simulink model "Hybrid2_modified"  (R2025a)
settings: Solver=FixedStepAuto  StartTime=0.0  StopTime=1.0  FixedStep=Ts  RelTol=1e-3
undefined symbols (not defined in the file or in its folder): closedLoop, controller, D1, D11, Delta, DiscIntNeverNeededParam, find_system, grid, level, protection, sensor, solarPanel, solarPlant, Ts
libraries: powerlib_extras x38, nesl_utility x29, spsSampleandHoldLib x24, spsThyristorLib x24, spsSeriesRLCBranchLib x23, simulink x22, fl_lib x18, ee_lib x12, spsEdgeDetectorLib x12, spsParallelRLCBranchLib x10, spsThreePhaseVIMeasurementLib x9, simulink_extras x8
(part 2 of 8)

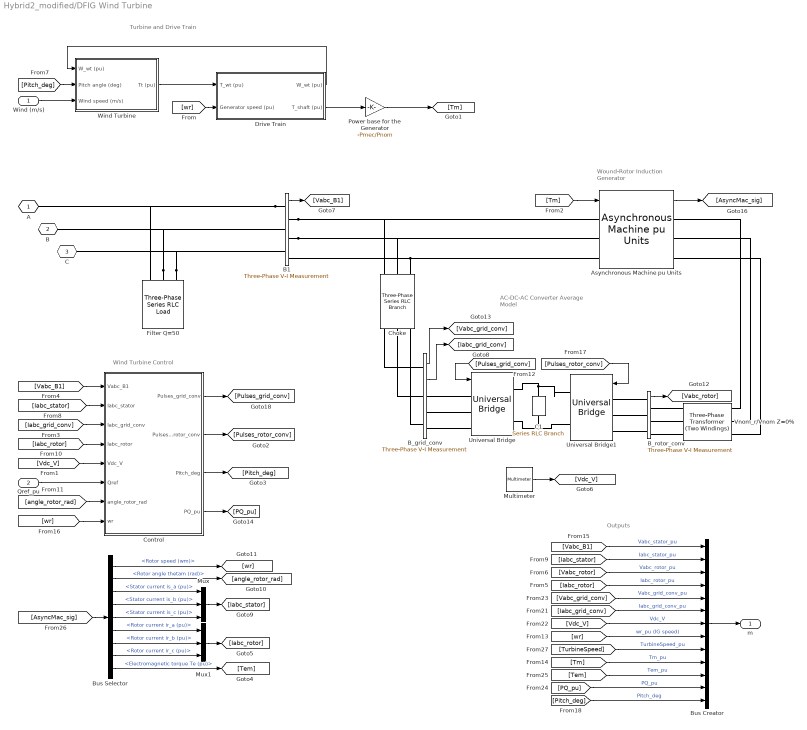
== system Hybrid2_modified/DFIG Wind Turbine ==
  note: Turbine and Drive Train
  note: Wind Turbine Control
  note: Wound-Rotor
      | Induction Generator
  note: AC-DC-AC Converter
      | Average Model
  note: Outputs
  "Wind (m/s) " : Inport
  Qref_pu : Inport  Port=2
  Asynchronous Machine pu Units : spsAsynchronousMachinepuUnitsLib/Asynchronous Machine pu Units  RotorType=Wound  PresetModel=No  MechanicalLoad=Torque Tm  ShowDetailedParameters=on  ReferenceFrame=Rotor  Units=pu  MeasurementBus=off  NominalParameters=[ Pnom Vnom Fnom ]  VoltageRatio=1  Stator=[ Rs Lls]  Rotor=[ Rr Llr]  Cage1=[0.01909 0.0397]  Cage2=[0.01909 0.0397]  Lm=Lm  Mechanical=[H F p]  PolePairs=3  InitialConditions=init  SimulateSaturation=off  Saturation="[0.212,0.4201,0.8125,1.0979,1.4799,2.2457,3.2586,4.5763,6.4763 ;   0.5,0.7,0.9,1,1.1,1.2 ,1.3,1.4,1.5]"  LoadFlowParameters=0  TsPowergui=0  TsBlock=-1  IterativeModel=Trapezoidal non iterative  IterativeDiscreteModel=Trapezoidal non iterative  Pmec=0
  B1 : spsThreePhaseVIMeasurementLib/Three-Phase V-I Measurement  VoltageMeasurement=phase-to-ground  SetLabelV=off  LabelV=Vabc  Vpu=on  VpuLL=off  CurrentMeasurement=no  SetLabelI=on  LabelI=Iabc_B1  Ipu=on  Pbase=Pnom  Vbase=Vnom  OutputType=Complex  PhasorSimulation=off  PSBequivalent=0
  B_grid_conv : spsThreePhaseVIMeasurementLib/Three-Phase V-I Measurement  VoltageMeasurement=phase-to-ground  SetLabelV=off  LabelV=Vabc_B1  Vpu=on  VpuLL=off  CurrentMeasurement=yes  SetLabelI=off  LabelI=Iabc  Ipu=on  Pbase=Pnom  Vbase=Vnom  OutputType=Complex  PhasorSimulation=off  PSBequivalent=0
  B_rotor_conv : spsThreePhaseVIMeasurementLib/Three-Phase V-I Measurement  VoltageMeasurement=phase-to-phase  SetLabelV=off  LabelV=Vabc_B1  Vpu=on  VpuLL=off  CurrentMeasurement=no  SetLabelI=off  LabelI=Iabc  Ipu=on  Pbase=Pnom  Vbase=Vnom_r  OutputType=Complex  PhasorSimulation=off  PSBequivalent=0
  Bus Creator : BusCreator  Inputs=13
  Bus Selector : BusSelector  OutputSignals=Mechanical.Rotor speed (wm),Mechanical.Rotor angle thetam (rad),Stator measurements.Stator current is_a (pu),Stator measurements.Stator current is_b (pu),Stator measurements.Stator current is_c (pu),Rotor measurements.Rotor current ir_a (pu),Rotor measurements.Rotor current ir_b (pu),Rotor measurements.Rotor current ir_c (pu),Mechanical.Electromagnetic torque Te (pu)
  C1 : spsSeriesRLCBranchLib/Series RLC Branch  LConnTagsString=__new0  RConnTagsString=__new0  BranchType=C  Resistance=[]  Inductance=[]  SetiL0=off  InitialCurrent=0  Capacitance=C_DClink  Setx0=on  InitialVoltage=Vdc_nom  Measurements=Branch voltage
  "Choke " : spsThreePhaseSeriesRLCBranchLib/Three-Phase Series RLC Branch  LConnTagsString=A|B|C  RConnTagsString=A|B|C  BranchType=RL  Resistance=R_RL*Vnom^2/Pnom  Inductance=L_RL*Vnom^2/Pnom/(2*pi*Fnom)  Capacitance=[]  Measurements=None
  Control : Subsystem
  Drive Train : Subsystem  mask(Wind Turbine shaft){H_WT=H_WT, Ksh=Ksh, D_mutual=D_mutual, wbase=2*pi*Fnom/p, w_wt0=w_wt0, torque0=torque0, Ts=Ts}
      mask prompts: H_WT "Wind turbine inertia constant H (s):"; Ksh "Shaft spring constant (pu of nominal mechanical torque/rad):"; D_mutual "Shaft mutual damping (pu of nominal mechanical torque/pu dw):"; wbase "Shaft base speed (rad/s):"; w_wt0 "Turbine initial speed (pu of base speed):"; torque0 "Initial output torque (pu of nominal mechanical torque):"; Ts "Sample time (s):"
      mask help:
      | This block implements a wind turbine drive train model. All shaft parameters are referred to high-speed shaft (generator shaft).
      |
      | The first input is the wind turbine torque in per unit (pu) based on the nominal power of the turbine and the base speed of the generator. The second input is the generator speed in pu based on the base speed of the generator.
      |
      | The outputs are:
      | 1- the transmitted torque of the shaft in pu based on the nominal power of the turbine and the base speed of the generator.
      | 2- the wind turbine speed in pu of the base speed of the generator.
  Filter Q=50 : spsThreePhaseSeriesRLCLoadLib/Three-Phase Series RLC Load  LConnTagsString=A|B|C  Configuration=Y (grounded)  NominalVoltage=Vnom  Vabc=[1e3 1e3 1e3]  Vabcp=[1e3 1e3 1e3]  NominalFrequency=Fnom  UnbalancedPower=off  ActivePower=C_var_filter/Q_filter  InductivePower=0  CapacitivePower=C_var_filter  Pabc=[10e3 9e3 11e3]  QLabc=[100 90 110]  QCabc=[100 90 110]  Pabcp=[10e3 9e3 11e3]  QLabcp=[100 90 110]  QCabcp=[100 90 110]  Measurements=None  LoadType=constant Z
  Multimeter : spsMultimeterLib/Multimeter  L=8  sel=1  yselected={}  Gain=1  OutputType=Complex  PlotAtSimulationStop=off  PhasorSimulation=off
  Mux : Mux  Inputs=3
  Mux1 : Mux  Inputs=3
  Power base for the Generator : Gain  Gain=-Pmec/Pnom  SaturateOnIntegerOverflow=on  OutDataTypeStr=Inherit: Same as input  ParamDataTypeStr=Inherit: Same as input
  Universal Bridge : spsUniversalBridgeLib/Universal Bridge  Arms=3  SnubberResistance=1e3  SnubberCapacitance=inf  Device=IGBT / Diodes  Ron=1e-4/Nb_wt  Lon=0  ForwardVoltages="[  0  0  ]"  ForwardVoltage=0  GTOparameters=[ 10e-6 , 20e-6 ]  IGBTparameters=[ 0 , 0 ]  Measurements=None  Measurements_2=None  converterType=Rectifier
  Universal Bridge1 : spsUniversalBridgeLib/Universal Bridge  Arms=3  SnubberResistance=1e3  SnubberCapacitance=inf  Device=IGBT / Diodes  Ron=1e-4/Nb_wt  Lon=0  ForwardVoltages="[  0  0  ]"  ForwardVoltage=0  GTOparameters=[ 10e-6 , 20e-6 ]  IGBTparameters=[ 0 , 0 ]  Measurements=None  Measurements_2=None  converterType=Rectifier
  Vnom_r/Vnom Z=0% : spsThreePhaseTransformerTwoWindingsLib/Three-Phase Transformer (Two Windings)  Winding1Connection=Y  Winding2Connection=Y  CoreType=Three single-phase transformers  SetSaturation=off  Hysteresis=off  DataFile='hysteresis'  SetInitialFlux=off  Measurements=None  UNITS=pu  NominalPower=[ Pnom , Fnom ]  Winding1=[ Vnom_r , 0, 0]  Winding2=[ Vnom , 0, 0]  Rm=500  Lm=inf  L0=0.5  Saturation=[ 0,0 ; 0.0024,1.2 ; 1.0,1.52 ]  InitialFluxes=[ 0.8 , -0.8 , 0.7 ]  BreakLoop=off  DiscreteSolver=Trapezoidal iterative  DataType=off  TransfoNumber=0
  Wind Turbine : Subsystem  mask(Wind Turbine){Prated=Pmec, c1_c8=c1_c8, K1_K2=K1_K2, wind0=wind0, Ts=Ts}
      mask prompts: Prated "Nominal mechanical output power (W):"; c1_c8 "Coefficients [c1 ... c8]"; K1_K2 "Parameters [K1 K2]"; wind0 "Initial wind speed (m/s):"; Ts "Sample time (s):"
      mask help:
      | This block implements a generic wind turbine models.
      |
      | The first input is the turbine speed in per unit of the generator base speed. For a synchronous or asynchronous generator, the base speed is the synchronous speed. For a permanent-magnet generator, the base speed is defined as the speed producing nominal voltage at  no load. The second input is the blade pitch angle in degrees. The third input is the wind speed in m/s.
      |
      | The output is the torque applied to the drive train in per unit based on the nominal power of the turbine and the base speed of the generator.
      mask init:
      | c1 = c1_c8(1);
      | c2 = c1_c8(2);
      | c3 = c1_c8(3);
      | c4 = c1_c8(4);
      | c5 = c1_c8(5);
      | c6 = c1_c8(6);
      | c7 = c1_c8(7);;
      | c8 = c1_c8(8);
      | 
      | K1=K1_K2(1);
      | K2=K1_K2(2);
      settings: OpenFcn=power_openblockproxy();
      mask Display: disp('');
  A : PMIOPort  Tag=PMCPort  Side=Left
  B : PMIOPort  Tag=PMCPort  Port=2  Side=Left
  C : PMIOPort  Tag=PMCPort  Port=3  Side=Left
  m : Outport  VectorParamsAs1DForOutWhenUnconnected=off
  wires:
  [Pulses_rotor_conv] -> Universal Bridge1/1
  [Pulses_grid_conv] -> Universal Bridge/1
  Multimeter/1 -> [Vdc_V]
  [Pitch_deg] -> Bus Creator/13  "Pitch_deg"
  [PQ_pu] -> Bus Creator/12  "PQ_pu"
  Control/4(PQ_pu) -> [PQ_pu]
  [Tem] -> Bus Creator/11  "Tem_pu"
  [Tm] -> Bus Creator/10  "Tm_pu"
  [TurbineSpeed] -> Bus Creator/9  "TurbineSpeed_pu"
  [Vdc_V] -> Bus Creator/7  "Vdc_V"
  [Iabc_grid_conv] -> Bus Creator/6  "Iabc_grid_conv_pu"
  [Vabc_grid_conv] -> Bus Creator/5  "Vabc_grid_conv_pu"
  [Iabc_rotor] -> Bus Creator/4  "Iabc_rotor_pu"
  [Vabc_rotor] -> Bus Creator/3  "Vabc_rotor_pu"
  [Iabc_stator] -> Bus Creator/2  "Iabc_stator_pu"
  [Vabc_B1] -> Bus Creator/1  "Vabc_stator_pu"
  Asynchronous Machine pu Units/1 -> [AsyncMac_sig]
  Control/2(Pulses_rotor_conv) -> [Pulses_rotor_conv]
  [Pitch_deg] -> Wind Turbine/2(Pitch angle (deg))
  Drive Train/1(W_wt (pu)) -> Wind Turbine/1(W_wt (pu))
  "Wind (m/s) "/1 -> Wind Turbine/3(Wind speed (m/s))
  Power base for the Generator/1 -> [Tm]
  Drive Train/2(T_shaft (pu)) -> Power base for the Generator/1
  [wr] -> Drive Train/2(Generator speed (pu))
  Wind Turbine/1(Tt (pu)) -> Drive Train/1(T_wt (pu))
  Qref_pu/1 -> Control/6(Qref)
  Bus Selector/9 -> [Tem]  "<Electromagnetic torque Te (pu)>"
  Bus Selector/1 -> [wr]  "<Rotor speed (wm)>"
  Bus Creator/1 -> m/1
  B_rotor_conv/1 -> [Vabc_rotor]
  B1/1 -> [Vabc_B1]
  [Vabc_B1] -> Control/1(Vabc_B1)
  [Iabc_grid_conv] -> Control/3(Iabc_grid_conv)
  [Iabc_rotor] -> Control/4(Iabc_rotor)
  [angle_rotor_rad] -> Control/7(angle_rotor_rad)
  Mux1/1 -> [Iabc_rotor]
  Mux/1 -> [Iabc_stator]
  [Vdc_V] -> Control/5(Vdc_V)
  Control/3(Pitch_deg) -> [Pitch_deg]
  [Iabc_stator] -> Control/2(Iabc_stator)
  [wr] -> Control/8(wr)
  Bus Selector/8 -> Mux1/3  "<Rotor current ir_c (pu)>"
  Bus Selector/7 -> Mux1/2  "<Rotor current ir_b (pu)>"
  Bus Selector/6 -> Mux1/1  "<Rotor current ir_a (pu)>"
  Bus Selector/5 -> Mux/3  "<Stator current is_c (pu)>"
  Bus Selector/4 -> Mux/2  "<Stator current is_b (pu)>"
  Bus Selector/3 -> Mux/1  "<Stator current is_a (pu)>"
  Bus Selector/2 -> [angle_rotor_rad]  "<Rotor angle thetam (rad)>"
  B_grid_conv/2 -> [Iabc_grid_conv]
  B_grid_conv/1 -> [Vabc_grid_conv]
  Control/1(Pulses_grid_conv) -> [Pulses_grid_conv]
  [AsyncMac_sig] -> Bus Selector/1
  [wr] -> Bus Creator/8  "wr_pu (IG speed)"
  [Tm] -> Asynchronous Machine pu Units/1
  connections:
  Universal Bridge1/LConn3 -- B_rotor_conv/LConn3
  Universal Bridge1/LConn2 -- B_rotor_conv/LConn2
  Universal Bridge1/LConn1 -- B_rotor_conv/LConn1
  C1/LConn1 -- Universal Bridge/RConn1 -- Universal Bridge1/RConn1
  B_grid_conv/RConn2 -- Universal Bridge/LConn2
  B_grid_conv/RConn1 -- Universal Bridge/LConn1
  B_grid_conv/RConn3 -- Universal Bridge/LConn3
  C1/RConn1 -- Universal Bridge/RConn2 -- Universal Bridge1/RConn2
  Filter Q=50/LConn3 -- B1/LConn3 -- C/RConn1
  Filter Q=50/LConn2 -- B1/LConn2 -- B/RConn1
  B1/LConn1 -- Filter Q=50/LConn1 -- A/RConn1
  B_rotor_conv/RConn3 -- Vnom_r/Vnom Z=0%/LConn3
  B_rotor_conv/RConn2 -- Vnom_r/Vnom Z=0%/LConn2
  B_rotor_conv/RConn1 -- Vnom_r/Vnom Z=0%/LConn1
  B1/RConn3 -- "Choke "/LConn3 -- Asynchronous Machine pu Units/LConn3
  B1/RConn1 -- "Choke "/LConn1 -- Asynchronous Machine pu Units/LConn1
  Asynchronous Machine pu Units/RConn3 -- Vnom_r/Vnom Z=0%/RConn3
  Asynchronous Machine pu Units/RConn1 -- Vnom_r/Vnom Z=0%/RConn1
  Asynchronous Machine pu Units/RConn2 -- Vnom_r/Vnom Z=0%/RConn2
  "Choke "/RConn3 -- B_grid_conv/LConn3
  "Choke "/RConn2 -- B_grid_conv/LConn2
  "Choke "/RConn1 -- B_grid_conv/LConn1
  B1/RConn2 -- "Choke "/LConn2 -- Asynchronous Machine pu Units/LConn2

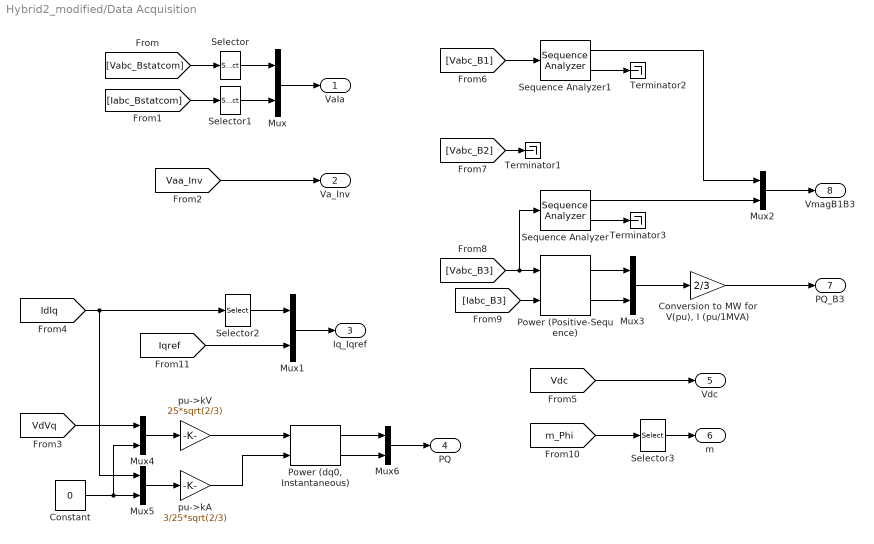
== system Hybrid2_modified/Data Acquisition ==
  Constant : Constant  Value=0
  "Conversion to MW for V(pu), I (pu/1MVA)" : Gain  Gain=2/3  SaturateOnIntegerOverflow=on  OutDataTypeStr=Inherit: Same as input  ParamDataTypeStr=Inherit: Same as input
  Mux{,1..3,6} (5 alike) : Mux  Inputs=2
  Mux4 : Mux  Inputs=[2,1]
  Mux5 : Mux  Inputs=[2,1]
  Power (Positive-Sequence) : spsPowerPositiveSequenceLib/Power (Positive-Sequence)  Freq=60  Vinit=[1, 0]  Iinit=[0, 0]  Ts=Ts
  "Power (dq0, Instantaneous)" : spsPowerdq0InstantaneousLib/Power (dq0, Instantaneous)
  Selector : Selector  InputPortWidth=3  IndexOptions=Index vector (dialog)  Indices=1  OutputSizes=1
  Selector1 : Selector  InputPortWidth=3  IndexOptions=Index vector (dialog)  Indices=1  OutputSizes=1
  Selector2 : Selector  InputPortWidth=2  IndexOptions=Index vector (dialog)  Indices=2  OutputSizes=1
  Selector3 : Selector  InputPortWidth=2  IndexOptions=Index vector (dialog)  Indices=1  OutputSizes=1
  Sequence Analyzer : spsSequenceAnalyzerLib/Sequence Analyzer  Freq=60  n=1  seq=Positive  InInit=[1, 0]  Ts=Ts
  Sequence Analyzer1 : spsSequenceAnalyzerLib/Sequence Analyzer  Freq=60  n=1  seq=Positive  InInit=[1, 0]  Ts=Ts
  Terminator1 : Terminator
  Terminator2 : Terminator
  Terminator3 : Terminator
  pu->kA : Gain  Gain=3/25*sqrt(2/3)  SaturateOnIntegerOverflow=on  OutDataTypeStr=Inherit: Same as input  ParamDataTypeStr=Inherit: Same as input
  pu->kV : Gain  Gain=25*sqrt(2/3)  SaturateOnIntegerOverflow=on  OutDataTypeStr=Inherit: Same as input  ParamDataTypeStr=Inherit: Same as input
  VaIa : Outport  VectorParamsAs1DForOutWhenUnconnected=off
  Va_Inv : Outport  Port=2  VectorParamsAs1DForOutWhenUnconnected=off
  Iq_Iqref : Outport  Port=3  VectorParamsAs1DForOutWhenUnconnected=off
  PQ : Outport  Port=4  VectorParamsAs1DForOutWhenUnconnected=off
  Vdc : Outport  Port=5  VectorParamsAs1DForOutWhenUnconnected=off
  m : Outport  Port=6  VectorParamsAs1DForOutWhenUnconnected=off
  PQ_B3 : Outport  Port=7  VectorParamsAs1DForOutWhenUnconnected=off
  VmagB1B3 : Outport  Port=8  VectorParamsAs1DForOutWhenUnconnected=off
  wires:
  [Vdc] -> Vdc/1
  Selector/1 -> Mux/1
  Selector1/1 -> Mux/2
  Mux/1 -> VaIa/1
  [m_Phi] -> Selector3/1
  [Vabc_Bstatcom] -> Selector/1
  [Iabc_Bstatcom] -> Selector1/1
  Mux1/1 -> Iq_Iqref/1
  Selector2/1 -> Mux1/1
  [Iqref] -> Mux1/2
  Selector3/1 -> m/1
  [Vaa_Inv] -> Va_Inv/1
  [Vabc_B2] -> Terminator1/1
  [Vabc_B1] -> Sequence Analyzer1/1
  Mux2/1 -> VmagB1B3/1
  Mux3/1 -> "Conversion to MW for V(pu), I (pu/1MVA)"/1
  Sequence Analyzer1/2 -> Terminator2/1
  Sequence Analyzer1/1 -> Mux2/1
  [Iabc_B3] -> Power (Positive-Sequence)/2
  [Vabc_B3] -> Sequence Analyzer/1, Power (Positive-Sequence)/1
  Sequence Analyzer/1 -> Mux2/2
  Power (Positive-Sequence)/1 -> Mux3/1
  Power (Positive-Sequence)/2 -> Mux3/2
  Sequence Analyzer/2 -> Terminator3/1
  "Conversion to MW for V(pu), I (pu/1MVA)"/1 -> PQ_B3/1
  pu->kV/1 -> "Power (dq0, Instantaneous)"/1
  pu->kA/1 -> "Power (dq0, Instantaneous)"/2
  [IdIq] -> Mux5/1, Selector2/1
  [VdVq] -> Mux4/1
  Mux4/1 -> pu->kV/1
  Mux5/1 -> pu->kA/1
  "Power (dq0, Instantaneous)"/1 -> Mux6/1
  "Power (dq0, Instantaneous)"/2 -> Mux6/2
  Mux6/1 -> PQ/1
  Constant/1 -> Mux5/2, Mux4/2

== system Hybrid2_modified/Distribution Statcom1 ==
  note: D-STATCOM
      | 25kV, +/- 3Mvar
      | Average Model
  note: +
  note: -
  note: -
  Bridge1 Average Model : spsUniversalBridgeLib/Universal Bridge  Arms=3  SnubberResistance=1e5  SnubberCapacitance=inf  Device=Average-model based VSC  Ron=1e-3  Lon=0  ForwardVoltages="[  0  0  ]"  ForwardVoltage=0  GTOparameters=[ 10e-6 , 20e-6 ]  IGBTparameters=[ 1e-6 , 2e-6 ]  Measurements=None  Measurements_2=None  converterType=Rectifier
  Bridge2 Average Model : spsUniversalBridgeLib/Universal Bridge  Arms=3  SnubberResistance=1e5  SnubberCapacitance=inf  Device=Average-model based VSC  Ron=1e-3  Lon=0  ForwardVoltages="[  0  0  ]"  ForwardVoltage=0  GTOparameters=[ 10e-6 , 20e-6 ]  IGBTparameters=[ 1e-6 , 2e-6 ]  Measurements=None  Measurements_2=None  converterType=Rectifier
  Ca_DVR : spsSeriesRLCBranchLib/Series RLC Branch  LConnTagsString=__new0  RConnTagsString=__new0  BranchType=RC  Resistance=100e-6*(2*pi*60)/40  Inductance=1.0  SetiL0=off  InitialCurrent=0  Capacitance=100e-6  Setx0=off  InitialVoltage=0  Measurements=None
  Ca_DVR1 : spsSeriesRLCBranchLib/Series RLC Branch  LConnTagsString=__new0  RConnTagsString=__new0  BranchType=RC  Resistance=100e-6*(2*pi*60)/40  Inductance=1.0  SetiL0=off  InitialCurrent=0  Capacitance=100e-6  Setx0=off  InitialVoltage=0  Measurements=None
  Ca_DVR2 : spsSeriesRLCBranchLib/Series RLC Branch  LConnTagsString=__new0  RConnTagsString=__new0  BranchType=RC  Resistance=100e-6*(2*pi*60)/40  Inductance=1.0  SetiL0=off  InitialCurrent=0  Capacitance=100e-6  Setx0=off  InitialVoltage=0  Measurements=None
  DC Link : spsParallelRLCBranchLib/Parallel RLC Branch  LConnTagsString=a  RConnTagsString=__new0  BranchType=C  Resistance=1.0  Inductance=1.0  SetiL0=off  InitialCurrent=0  Capacitance=10000e-6  Setx0=off  InitialVoltage=0  Measurements=None
  D_statcom_avg Controller : Subsystem  mask(D-STATCOM Controller){ModeOper=Voltage regulation, Vac_Ref=1.0, Qref=0, Vdc_Ref=2400, Par_VacReg=[0.55 2500], Par_VdcReg=[0.001 0.15], Par_IReg=[0.8 200 0], Ts=2e-4}
      mask prompts: ModeOper "Mode of operation:"; Vac_Ref "AC voltage setpoint Vref (pu):"; Qref "Manual mode: Qref (Reactive power in pu):"; Vdc_Ref "DC Voltage setpoint (Volts)"; Par_VacReg "Vac Regulator Gains: [ Kp  Ki ]"; Par_VdcReg "Vdc Regulator Gains: [ Kp  Ki ]"; Par_IReg "Current Regulators Gain: [ Kp Ki Kd ]"; Ts "Sample time (s)"
      mask init:
      | Kp_I=Par_IReg(1);
      | Ki_I=Par_IReg(2);
      | Kd_I=Par_IReg(3);
      | Kp_Vdc=Par_VdcReg(1);
      | Ki_Vdc=Par_VdcReg(2);
      | Kp_Vac=Par_VacReg(1);
      | Ki_Vac=Par_VacReg(2);
      mask TypeOptions ModeOper: Voltage regulation | Q regulation
  Gain : Gain  Gain=-1
  Ground : spsGroundLib/Ground  LConnTagsString=a
  Ground1 : spsGroundLib/Ground  LConnTagsString=a
  Ground2 : spsGroundLib/Ground  LConnTagsString=a
  La_DVR : spsSeriesRLCBranchLib/Series RLC Branch  LConnTagsString=__new0  RConnTagsString=__new0  BranchType=L  Resistance=1.0  Inductance=800e-6  SetiL0=off  InitialCurrent=0  Capacitance=1.0  Setx0=off  InitialVoltage=0  Measurements=None
  La_DVR1 : spsSeriesRLCBranchLib/Series RLC Branch  LConnTagsString=__new0  RConnTagsString=__new0  BranchType=L  Resistance=1.0  Inductance=800e-6  SetiL0=off  InitialCurrent=0  Capacitance=1.0  Setx0=off  InitialVoltage=0  Measurements=None
  La_DVR2 : spsSeriesRLCBranchLib/Series RLC Branch  LConnTagsString=__new0  RConnTagsString=__new0  BranchType=L  Resistance=1.0  Inductance=800e-6  SetiL0=off  InitialCurrent=0  Capacitance=1.0  Setx0=off  InitialVoltage=0  Measurements=None
  Tr A : spsLinearTransformerLib/Linear Transformer  UNITS=pu  NominalPower=[3e6/3 60]  winding1=[1250 0.03/30 0.03]  winding2=[25e3/sqrt(3) 0.03/30 0.03]  ThreeWindings=off  winding3=[60e3 0.005 0.02]  RmLm=[200 200]  Measurements=None  DataType=off
  Tr B : spsLinearTransformerLib/Linear Transformer  UNITS=pu  NominalPower=[3e6/3 60]  winding1=[1250 0.03/30 0.03]  winding2=[25e3/sqrt(3) 0.03/30 0.03]  ThreeWindings=off  winding3=[60e3 0.005 0.02]  RmLm=[200 200]  Measurements=None  DataType=off
  Tr C : spsLinearTransformerLib/Linear Transformer  UNITS=pu  NominalPower=[3e6/3 60]  winding1=[1250 0.03/30 0.03]  winding2=[25e3/sqrt(3) 0.03/30 0.03]  ThreeWindings=off  winding3=[60e3 0.005 0.02]  RmLm=[200 200]  Measurements=None  DataType=off
  Voltage Measurement : spsVoltageMeasurementLib/Voltage Measurement  Tag=PoWeRsYsTeMmEaSuReMeNt  PhasorSimulation=off  OutputType=Magnitude  PSBequivalent=0
  Voltage Measurement1 : spsVoltageMeasurementLib/Voltage Measurement  Tag=PoWeRsYsTeMmEaSuReMeNt  PhasorSimulation=off  OutputType=Magnitude  PSBequivalent=0
  A : PMIOPort  Side=Right
  B : PMIOPort  Port=2  Side=Right
  C : PMIOPort  Port=3  Side=Right
  tag scope: Vaa_Inv=global, Vdc_Statcom=global
  wires:
  [Vabc_Bstatcom] -> D_statcom_avg Controller/2(Vabc)
  [Iabc_Bstatcom] -> D_statcom_avg Controller/3(Iabc)
  Voltage Measurement/1 -> [Vdc_Statcom]
  [Vdc] -> D_statcom_avg Controller/1(Vdc)
  D_statcom_avg Controller/1(Vref_abc) -> Bridge1 Average Model/1, Gain/1
  Gain/1 -> Bridge2 Average Model/1
  Voltage Measurement1/1 -> [Vaa_Inv]
  connections:
  Bridge2 Average Model/LConn2 -- Ca_DVR1/LConn1 -- Tr B/LConn2
  Tr C/LConn2 -- Ca_DVR2/LConn1 -- Bridge2 Average Model/LConn3
  Ca_DVR1/RConn1 -- La_DVR1/RConn1 -- Tr B/LConn1
  Ca_DVR2/RConn1 -- La_DVR2/RConn1 -- Tr C/LConn1
  Tr A/LConn1 -- La_DVR/RConn1 -- Ca_DVR/RConn1
  Tr C/RConn2 -- Ground2/LConn1
  Tr B/RConn2 -- Ground1/LConn1
  Tr A/RConn2 -- Ground/LConn1
  A/RConn1 -- Tr A/RConn1
  Tr B/RConn1 -- B/RConn1
  C/RConn1 -- Tr C/RConn1
  Tr A/LConn2 -- Ca_DVR/LConn1 -- Bridge2 Average Model/LConn1 -- Voltage Measurement1/LConn2
  Bridge1 Average Model/RConn1 -- Bridge2 Average Model/RConn1 -- DC Link/LConn1 -- Voltage Measurement/LConn1
  Bridge1 Average Model/LConn1 -- La_DVR/LConn1 -- Voltage Measurement1/LConn1
  Bridge1 Average Model/LConn2 -- La_DVR1/LConn1
  Bridge1 Average Model/LConn3 -- La_DVR2/LConn1
  DC Link/RConn1 -- Bridge1 Average Model/RConn2 -- Bridge2 Average Model/RConn2 -- Voltage Measurement/LConn2

== system Hybrid2_modified/Filter & AC Measurements ==
  Current Sensor Dynamics : Subsystem
  Current Sensor1 : ee_lib/Sensors & Transducers/Current Sensor (Three-Phase)
  Neutral Port (Three-Phase) : ee_lib/Connectors & References/Neutral Port (Three-Phase)  G_parasitic=1e-12 1/Ohm
      settings: InternalSimscapePortConfiguration="{\"Bottom\":[],\"Left\":[{\"id\":\"N\",\"label\":\"~\",\"type\":\"foundation.electrical.three_phase\"}],\"Right\":[{\"id\":\"n\",\"label\":\"n\",\"type\":\"foundation.electrical.electrical\"}],\"Top\":[]}"
  PS-Simulink Converter : nesl_utility/PS-Simulink Converter  PhysicalDomain=network_engine_domain  SubClassName=ps_output  LeftPortType=input  RightPortType=output  PseudoPeriodic=off  Frequencies=[]  VectorFormat=1-D array  Unit=inherit  AffineConversion=off
  PS-Simulink Converter1 : nesl_utility/PS-Simulink Converter  PhysicalDomain=network_engine_domain  SubClassName=ps_output  LeftPortType=input  RightPortType=output  PseudoPeriodic=off  Frequencies=[]  VectorFormat=1-D array  Unit=inherit  AffineConversion=off
  Phase Voltage Sensor (Three-Phase) : ee_lib/Sensors & Transducers/Phase Voltage Sensor (Three-Phase)
  RLC (Three-Phase) : ee_lib/Passive/RLC Assemblies/RLC (Three-Phase)  port_option=ee.enum.threePhasePort.composite  component_structure=4  R=solarPlant.inductorResistance Ohm  L=solarPlant.lineInductance H  C=1e-6 F  R_parasitic=1e-6 Ohm  G_parasitic=1e-6 1/Ohm  IL_specify=on  IL_priority=High  IL=[0, 0, 0] A  IL_nominal_specify=off  IL_nominal_value=1  IL_nominal_unit=A  VC_specify=on  VC_priority=High  VC=[0, 0, 0] V  VC_nominal_specify=off  VC_nominal_value=1  VC_nominal_unit=V
      settings: InternalSimscapePortConfiguration="{\"Bottom\":[],\"Left\":[{\"id\":\"N1\",\"label\":\"~1\",\"type\":\"foundation.electrical.three_phase\"}],\"Right\":[{\"id\":\"N2\",\"label\":\"~2\",\"type\":\"foundation.electrical.three_phase\"}],\"Top\":[]}"
  Scope : Scope  NumInputPorts=2
      settings: ActiveDisplayYMinimum=-169.31893  ActiveDisplayYMaximum=165.34576
  Voltage Sensor Dynamics : Subsystem
  ABC1 : PMIOPort  Side=Left
  ABC2 : PMIOPort  Port=2  Side=Right
  N : PMIOPort  Port=3  Side=Right
  Iabc : Outport
  Vabc : Outport  Port=2
  wires:
  PS-Simulink Converter/1 -> Scope/1, Current Sensor Dynamics/1(Iabc1)
  Current Sensor Dynamics/1(Iabc2) -> Iabc/1
  Voltage Sensor Dynamics/1(Vabc2) -> Vabc/1
  PS-Simulink Converter1/1 -> Scope/2, Voltage Sensor Dynamics/1(Vabc1)
  connections:
  Current Sensor1/LConn1 -- RLC (Three-Phase)/RConn1
  Phase Voltage Sensor (Three-Phase)/LConn1 -- ABC2/RConn1 -- Current Sensor1/RConn2
  PS-Simulink Converter/LConn1 -- Current Sensor1/RConn1
  PS-Simulink Converter1/LConn1 -- Phase Voltage Sensor (Three-Phase)/RConn1
  Neutral Port (Three-Phase)/LConn1 -- Phase Voltage Sensor (Three-Phase)/RConn2
  Neutral Port (Three-Phase)/RConn1 -- N/RConn1
  RLC (Three-Phase)/LConn1 -- ABC1/RConn1

== system Hybrid2_modified/Grid ==
  Resistor : fl_lib/Electrical/Electrical Elements/Resistor  R=50 Ohm  i_specify=off  i_priority=None  i=0 A  i_nominal_specify=off  i_nominal_value=1  i_nominal_unit=A  v_specify=off  v_priority=None  v=0 V  v_nominal_specify=off  v_nominal_value=1  v_nominal_unit=V
  Voltage Source (Three-Phase) : ee_lib/Sources/Voltage Source (Three-Phase)  vline_rms=grid.actualLineVoltage V  shift=0 deg  freq=grid.frequency Hz  impedance_option=0  SShortCircuit=1e6 V*A  XR=15  R=0.01 Ohm  L=3.97e-4 H  harmonic_option=0  harmonic_orders=[5, 7, 11, 13]  harmonic_ratios=[.1, .1, .1, .1]  G_parasitic=0 1/Ohm  I_specify=off  I_priority=None  I=[ 0 0 0 ] A  I_nominal_specify=off  I_nominal_value=1  I_nominal_unit=A
  ABC : PMIOPort  Side=Left
  N : PMIOPort  Port=2  Side=Left
  E : PMIOPort  Port=3  Side=Left
  connections:
  E/RConn1 -- Resistor/RConn1
  ABC/RConn1 -- Voltage Source (Three-Phase)/RConn1
  Voltage Source (Three-Phase)/LConn1 -- N/RConn1 -- Resistor/LConn1

== system Hybrid2_modified/Linearization I//O points ==
  u2 : Inport
  u1 : Inport  Port=2
  "Set to 1 for closed-loop operation, and set to 0 when linearizing" : Gain  Gain=closedLoop  SaturateOnIntegerOverflow=on  OutDataTypeStr=Inherit: Same as input  ParamDataTypeStr=Inherit: Same as input
  Sum1 : Sum  Inputs=++|  InputSameDT=on  SaturateOnIntegerOverflow=on  OutDataTypeStr=Inherit: Same as first input
  y2 : Outport  VectorParamsAs1DForOutWhenUnconnected=off
  y1 : Outport  Port=2  VectorParamsAs1DForOutWhenUnconnected=off
  wires:
  Sum1/1 -> y1/1
  u2/1 -> Sum1/1
  "Set to 1 for closed-loop operation, and set to 0 when linearizing"/1 -> Sum1/2
  u1/1 -> y2/1, "Set to 1 for closed-loop operation, and set to 0 when linearizing"/1

== system Hybrid2_modified/MPPT ==
  Ipv : Inport
  Vpv : Inport  Port=2
  Constant : Constant  Value=solarPlant.endMPPTValue
  MPPT Algorithm : Subsystem  Variant=on
  Switch : Switch  Threshold=solarPlant.endMPPTValue  SaturateOnIntegerOverflow=off  InputSameDT=off
  Vmpp : Outport  VectorParamsAs1DForOutWhenUnconnected=off
  tag scope: Ipvnow=global, Vpvnow=global
  wires:
  Vpv/1 -> [Vpvnow], MPPT Algorithm/2(Vpv)
  Ipv/1 -> [Ipvnow], MPPT Algorithm/1(Ipv)
  Constant/1 -> Switch/1
  MPPT Algorithm/1(Vmpp) -> Switch/3, Switch/2
  Switch/1 -> Vmpp/1

== system Hybrid2_modified/Modulation Signal ==
  Vd : Inport
  Vq : Inport  Port=2
  Angle : Inport  Port=3
  Vdc : Inport  Port=4
  Gating Signal : Subsystem
  "dq to alpha beta " : Subsystem
  mabc : Outport  VectorParamsAs1DForOutWhenUnconnected=off
  wires:
  Gating Signal/1(mabc) -> mabc/1
  Vdc/1 -> Gating Signal/2(Vdc)
  "dq to alpha beta "/1(Vabc) -> Gating Signal/1(Vmod)
  Vd/1 -> "dq to alpha beta "/1("d ")
  Angle/1 -> "dq to alpha beta "/3(angle)
  Vq/1 -> "dq to alpha beta "/2(q)

== system Hybrid2_modified/PLL and Protection ==
  Vabc : Inport
  Vpv : Inport  Port=2
  Iabc : Inport  Port=3
  Constant : Constant  Value=pi/2
  Gain2 : Gain  Gain=2*pi
  Protection : Subsystem
  "Sinusoidal Measurement (PLL, Three-Phase)" : eeSinusoidalMeasurement/Sinusoidal Measurement (PLL, Three-Phase)  Kp_LF=0.05  Ki_LF=1  F0=grid.frequency  Theta0=0  Ts=0
  Subtract : Sum  Inputs=-+
  Vphm to Vsd : Gain  Gain=3/2
  w : Outport  VectorParamsAs1DForOutWhenUnconnected=off
  angle : Outport  Port=2  VectorParamsAs1DForOutWhenUnconnected=off
  Vsd : Outport  Port=3  VectorParamsAs1DForOutWhenUnconnected=off
  TripSig : Outport  Port=4  VectorParamsAs1DForOutWhenUnconnected=off
  wires:
  "Sinusoidal Measurement (PLL, Three-Phase)"/3 -> Vphm to Vsd/1
  Gain2/1 -> Protection/1(w), w/1
  "Sinusoidal Measurement (PLL, Three-Phase)"/1 -> Gain2/1
  Vabc/1 -> "Sinusoidal Measurement (PLL, Three-Phase)"/1
  Protection/1(TS) -> TripSig/1
  Vpv/1 -> Protection/3(Vpv)
  Iabc/1 -> Protection/4(Iac)
  Subtract/1 -> angle/1
  "Sinusoidal Measurement (PLL, Three-Phase)"/2 -> Subtract/2
  Constant/1 -> Subtract/1
  Vphm to Vsd/1 -> Vsd/1, Protection/2(Vsd)

== system Hybrid2_modified/Power Circuit ==
  note: Solar panel parasitic capacitance
  note: Solar panel parasitic capacitance
  C1 : fl_lib/Electrical/Electrical Elements/Capacitor  c=solarPlant.capacitance*2 F  r=1e-6 Ohm  g=0 1/Ohm  i_specify=off  i_priority=High  i=0 A  i_nominal_specify=off  i_nominal_value=1  i_nominal_unit=A  v_specify=off  v_priority=High  v=0 V  v_nominal_specify=off  v_nominal_value=1  v_nominal_unit=V  vc_specify=on  vc_priority=High  vc=solarPlant.DCMPPTValue/2 V  vc_nominal_specify=off  vc_nominal_value=1  vc_nominal_unit=V
  C2 : fl_lib/Electrical/Electrical Elements/Capacitor  c=solarPlant.capacitance*2 F  r=1e-6 Ohm  g=0 1/Ohm  i_specify=off  i_priority=High  i=0 A  i_nominal_specify=off  i_nominal_value=1  i_nominal_unit=A  v_specify=off  v_priority=High  v=0 V  v_nominal_specify=off  v_nominal_value=1  v_nominal_unit=V  vc_specify=on  vc_priority=High  vc=solarPlant.DCMPPTValue/2 V  vc_nominal_specify=off  vc_nominal_value=1  vc_nominal_unit=V
  C3 : fl_lib/Electrical/Electrical Elements/Capacitor  c=solarPlant.parasiticCapacitance/2 F  r=1 Ohm  g=0 1/Ohm  i_specify=off  i_priority=High  i=0 A  i_nominal_specify=off  i_nominal_value=1  i_nominal_unit=A  v_specify=off  v_priority=High  v=0 V  v_nominal_specify=off  v_nominal_value=1  v_nominal_unit=V  vc_specify=on  vc_priority=High  vc=solarPlant.DCMPPTValue V  vc_nominal_specify=off  vc_nominal_value=1  vc_nominal_unit=V
  C4 : fl_lib/Electrical/Electrical Elements/Capacitor  c=solarPlant.parasiticCapacitance/2 F  r=1 Ohm  g=0 1/Ohm  i_specify=off  i_priority=High  i=0 A  i_nominal_specify=off  i_nominal_value=1  i_nominal_unit=A  v_specify=off  v_priority=High  v=0 V  v_nominal_specify=off  v_nominal_value=1  v_nominal_unit=V  vc_specify=on  vc_priority=High  vc=solarPlant.DCMPPTValue V  vc_nominal_specify=off  vc_nominal_value=1  vc_nominal_unit=V
  DC Current Sensor : Subsystem
      mask Display: disp('i')
  DC Voltage Sensor : Subsystem
      mask Display: disp('v');
  Power Circuit : Subsystem  Variant=on  VariantControl=Variant1
  + : PMIOPort  Side=Left
  - : PMIOPort  Port=2  Side=Left
  ABC : PMIOPort  Port=3  Side=Right
  E : PMIOPort  Port=4  Side=Right
  wires:
  [mABC] -> Power Circuit/1(m)
  [TripSig] -> Power Circuit/2(TripSig)
  connections:
  -/RConn1 -- DC Voltage Sensor/LConn1 -- C4/LConn1 -- Power Circuit/LConn3 -- C2/RConn1
  C2/LConn1 -- Power Circuit/LConn2 -- C1/RConn1
  DC Current Sensor/LConn1 -- C3/LConn1 -- Power Circuit/LConn1 -- C1/LConn1 -- DC Voltage Sensor/RConn1
  DC Current Sensor/RConn1 -- +/RConn1
  C3/RConn1 -- E/RConn1 -- C4/RConn1
  ABC/RConn1 -- Power Circuit/RConn1

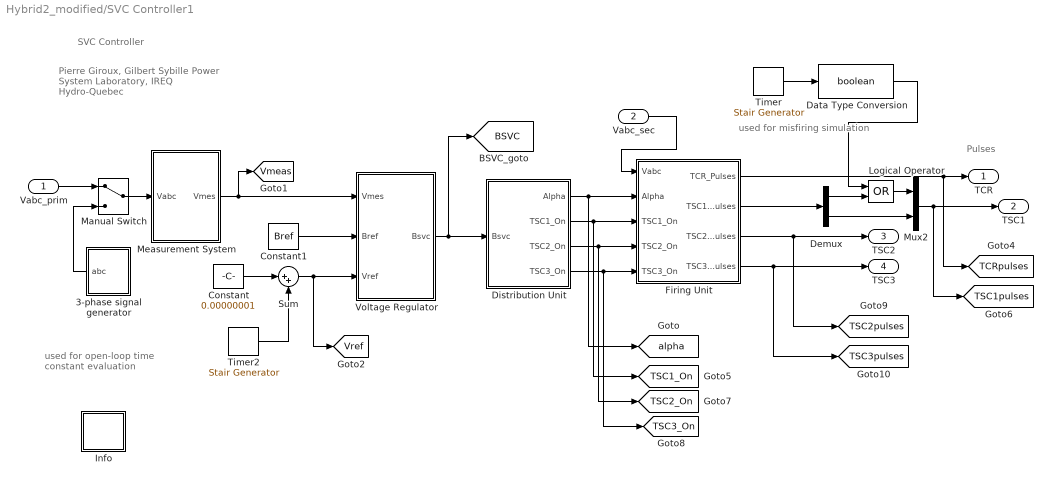
== system Hybrid2_modified/SVC Controller1 ==
  note: Pulses
  note: SVC Controller
  note: Pierre Giroux, Gilbert Sybille
      | Power System Laboratory, IREQ
      | Hydro-Quebec
  note: used for misfiring
      | simulation
  note: used for open-loop
      | time constant evaluation
  Vabc_prim : Inport  PortDimensions=3
  Vabc_sec : Inport  Port=2  PortDimensions=3
  3-phase signal generator : Subsystem
  Constant : Constant  Value=0.00000001
  Constant1 : Constant  Value=Bref
  Data Type Conversion : DataTypeConversion  OutDataTypeStr=boolean  SaturateOnIntegerOverflow=off  RndMeth=Floor
  Demux : Demux  Outputs=[1 5]
      settings: DisplayOption=none
  Distribution Unit : Subsystem  mask(Distribution Unit){ParNom=[333e6 60], Xf_xfo=0.15, Vsec_svc=16e3, L_TCR=18.7e-3, C_TSC=308.4e-6, L_TSC=1.13e-3, hyst_svc=0.1, Ts=Ts}
      mask prompts: ParNom "Transformer nominal power and frequency: [  P (VA)    Freq (Hz)  ]"; Xf_xfo "Transformer total leakage (pu/Pnom):"; Vsec_svc "Nominal secondary voltage (Volts rms ph-ph):"; L_TCR "TCR branch inductance (H):"; C_TSC "TSC branch capacitance (F):"; L_TSC "TSC branch inductance (H)"; hyst_svc "Hysteresis - Distribution unit (pu/100MVA):"; Ts "Sample time:"
      mask init:
      | Pnom_xfo=ParNom(1);
      | Freq=ParNom(2);
      | Bsec_pu100=100e6/Vsec_svc/Vsec_svc/3;
      | w=2*pi*Freq;
      | Bpu_TCR=-1/L_TCR/w/Bsec_pu100;
      | Bpu_TSC=1/(1/w/C_TSC-L_TSC*w)/Bsec_pu100;
      | B=1:-0.0025:0.0;
      | B=B';
      | for i=1:401,
      |       if B(i) <= 0,
      | 	ang = 0;
      |       elseif B(i) >= 1,
      | 	ang = pi;
      |       else,
      | 	a = pi; e = .0001;
      | 	da = a;
      | 	while abs(da)>e,
      | 		da = (pi*B(i)-a+sin(a))/(1-cos(a));
      | 		a = a + da;
      | 	end;
      | 	ang = a;
      |       end;
      |       A(i)=(180-ang*180/pi)/2+90;
      | end
      | A=A';
      | B=-B;
  Firing Unit : Subsystem  mask(Firing Unit){FiringMode=Synchronized, Nstep=0, ParInit=[0 60], Ts=Ts}
      mask prompts: FiringMode "Firing mode"; Nstep "Total delay (in number of time step)"; ParInit "Initial phase and frequency of input: [ Phase (degree)  Freq (Hz) ]"; Ts "Sample time:"
      mask init:
      | PhaseInit=ParInit(1);
      | FreqInit=ParInit(2);
      mask TypeOptions FiringMode: Synchronized | Continuous
  Info : Subsystem
      mask Display: disp('?')
  Logical Operator : Logic  Operator=OR
  Manual Switch : ManualSwitch
  Measurement System : Subsystem  mask(SVC measurement system){Vnom=735e3, ParI=[735e3*0.9998 0 60], Ts=Ts}
      mask prompts: Vnom "Nominal voltage (volts rms ph-ph)"; ParI "Initial input: [ Mag (volts rms ph-ph)  Phase (degree) Freq (Hz) ]"; Ts "Sample time:"
      mask init:
      | Mag_Init=ParI(1)/Vnom;
      | Phase_Init=ParI(2);
      | Freq_Init=ParI(3);
  Mux2 : Mux  Inputs=[1 5]
  Sum : Sum  Inputs=|++  SaturateOnIntegerOverflow=on
  Timer : spsStairGeneratorLib/Stair Generator  t="[ 0  0.121  0.121+eps ]*100"  e="[0  1  0 ]"  Ts=Ts
  Timer2 : spsStairGeneratorLib/Stair Generator  t="[ 0  0.4  0.6 ]"  e=[1 1 1 ]  Ts=Ts
  Voltage Regulator : Subsystem
  TCR : Outport  VectorParamsAs1DForOutWhenUnconnected=off
  TSC1 : Outport  Port=2  VectorParamsAs1DForOutWhenUnconnected=off
  TSC2 : Outport  Port=3  VectorParamsAs1DForOutWhenUnconnected=off
  TSC3 : Outport  Port=4  VectorParamsAs1DForOutWhenUnconnected=off
  tag scope: BSVC=global, TCRpulses=global, TSC1_On=global, TSC1pulses=global, TSC2_On=global, TSC2pulses=global, TSC3_On=global, TSC3pulses=global, Vmeas=global, Vref=global, alpha=global
  wires:
  Firing Unit/2(TSC1_Pulses) -> Demux/1
  Measurement System/1(Vmes) -> Voltage Regulator/1(Vmes), [Vmeas]
  Constant1/1 -> Voltage Regulator/2(Bref)
  Mux2/1 -> TSC1/1, [TSC1pulses]
  Demux/2 -> Mux2/2
  Logical Operator/1 -> Mux2/1
  Demux/1 -> Logical Operator/2
  Voltage Regulator/1(Bsvc) -> Distribution Unit/1(Bsvc), [BSVC]
  Sum/1 -> [Vref], Voltage Regulator/3(Vref)
  Constant/1 -> Sum/1
  Vabc_prim/1 -> Manual Switch/1
  Manual Switch/1 -> Measurement System/1(Vabc)
  3-phase signal generator/1(abc) -> Manual Switch/2
  Firing Unit/1(TCR_Pulses) -> TCR/1, [TCRpulses]
  Firing Unit/3(TSC2_Pulses) -> TSC2/1, [TSC2pulses]
  Firing Unit/4(TSC3_Pulses) -> TSC3/1, [TSC3pulses]
  Distribution Unit/1(Alpha) -> Firing Unit/2(Alpha), [alpha]
  Distribution Unit/2(TSC1_On) -> Firing Unit/3(TSC1_On), [TSC1_On]
  Distribution Unit/3(TSC2_On) -> Firing Unit/4(TSC2_On), [TSC2_On]
  Distribution Unit/4(TSC3_On) -> Firing Unit/5(TSC3_On), [TSC3_On]
  Vabc_sec/1 -> Firing Unit/1(Vabc)
  Timer2/1 -> Sum/2
  Timer/1 -> Data Type Conversion/1
  Data Type Conversion/1 -> Logical Operator/1

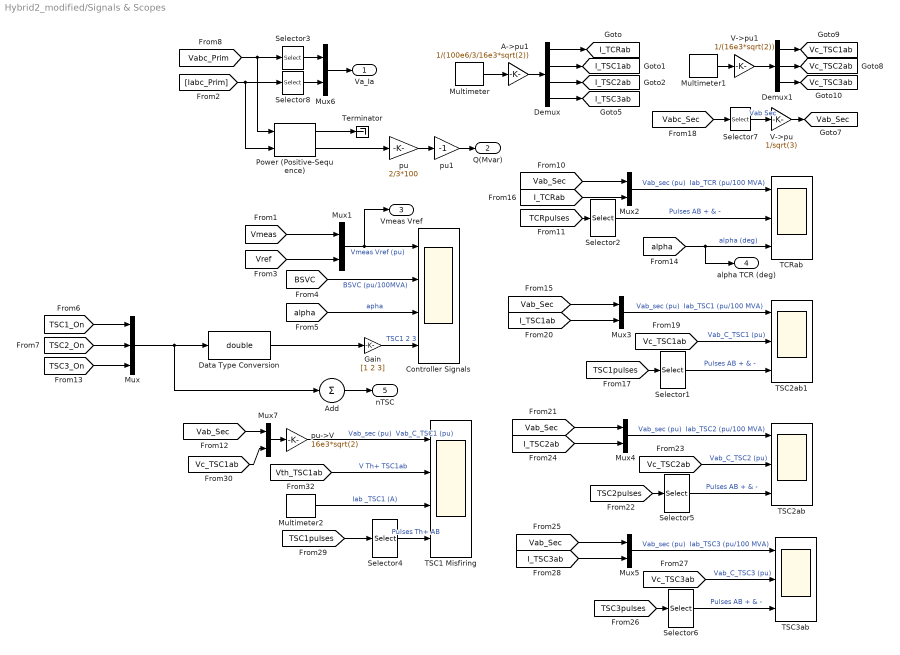
== system Hybrid2_modified/Signals & Scopes ==
  A->pu1 : Gain  Gain=1/(100e6/3/16e3*sqrt(2))  SaturateOnIntegerOverflow=on  OutDataTypeStr=Inherit: Same as input  ParamDataTypeStr=Inherit: Same as input
  Add : Sum  Inputs=+
  Controller Signals : Scope  NumInputPorts=4
      settings: SampleTime=Ts  ActiveDisplayYMinimum=0.92  ActiveDisplayYMaximum=1.04  DataLoggingVariableName=Ctrl_Sig  DataLoggingSaveFormat=Array
  Data Type Conversion : DataTypeConversion  OutDataTypeStr=double  SaturateOnIntegerOverflow=off  RndMeth=Floor
  Demux : Demux
      settings: DisplayOption=none
  Demux1 : Demux  Outputs=3
      settings: DisplayOption=none
  Gain : Gain  Gain=[1 2 3]  OutDataTypeStr=double  SaturateOnIntegerOverflow=on  ParamDataTypeStr=Inherit: Same as input
  Multimeter : spsMultimeterLib/Multimeter  Tag=PoWeRsYsTeMmEaSuReMeNt  L=8  sel=[4 5 6 7]  yselected={}  Gain=[1 1 1 1]  OutputType=Magnitude  PlotAtSimulationStop=off  PhasorSimulation=off
      settings: AttributesFormatString=\n
  Multimeter1 : spsMultimeterLib/Multimeter  Tag=PoWeRsYsTeMmEaSuReMeNt  L=8  sel=[1 2 3]  yselected={}  Gain=[1 1 1]  OutputType=Magnitude  PlotAtSimulationStop=off  PhasorSimulation=off
      settings: AttributesFormatString=\n
  Multimeter2 : spsMultimeterLib/Multimeter  Tag=PoWeRsYsTeMmEaSuReMeNt  L=8  sel=5  yselected={}  Gain=1  OutputType=Magnitude  PlotAtSimulationStop=off  PhasorSimulation=off
      settings: AttributesFormatString=\n
  Mux : Mux  Inputs=3
  Mux{1..7} (7 alike) : Mux  Inputs=2
  Power (Positive-Sequence) : spsPowerPositiveSequenceLib/Power (Positive-Sequence)  Freq=60  Vinit=[1 0]  Iinit=[0.05 90]  Ts=Ts
  Selector{1..2,5..6} (4 alike) : Selector  InputPortWidth=6  IndexOptions=Index vector (dialog)  Indices=[1 2]  OutputSizes=1
  Selector3 : Selector  InputPortWidth=3  IndexOptions=Index vector (dialog)  Indices=1  OutputSizes=1
  Selector4 : Selector  InputPortWidth=6  IndexOptions=Index vector (dialog)  Indices=[1 ]  OutputSizes=1
  Selector7 : Selector  InputPortWidth=3  IndexOptions=Index vector (dialog)  Indices=1  OutputSizes=1
  Selector8 : Selector  InputPortWidth=3  IndexOptions=Index vector (dialog)  Indices=1  OutputSizes=1
  TCRab : Scope  NumInputPorts=3
      settings: SampleTime=Ts  TimeSpan=0.04  ActiveDisplayYMinimum=-1.75  ActiveDisplayYMaximum=1.75  DataLoggingVariableName=VI_TCRab
  TSC1 Misfiring : Scope  NumInputPorts=4
      settings: SampleTime=Ts  TimeSpan=0.35  ActiveDisplayYMinimum=-30000  ActiveDisplayYMaximum=30000  DataLoggingVariableName=VI_TCRab4
  TSC2ab : Scope  NumInputPorts=3
      settings: SampleTime=Ts  TimeSpan=0.04  ActiveDisplayYMinimum=-2  ActiveDisplayYMaximum=2  DataLoggingVariableName=VI_TCRab2
  TSC2ab1 : Scope  NumInputPorts=3
      settings: SampleTime=Ts  TimeSpan=0.04  ActiveDisplayYMinimum=-2  ActiveDisplayYMaximum=2  DataLoggingVariableName=VI_TCRab1
  TSC3ab : Scope  NumInputPorts=3
      settings: SampleTime=Ts  TimeSpan=0.04  ActiveDisplayYMinimum=-2  ActiveDisplayYMaximum=2  DataLoggingVariableName=VI_TCRab3
  Terminator : Terminator
  "V->pu " : Gain  Gain=1/sqrt(3)  SaturateOnIntegerOverflow=on  OutDataTypeStr=Inherit: Same as input  ParamDataTypeStr=Inherit: Same as input
  V->pu1 : Gain  Gain=1/(16e3*sqrt(2))  SaturateOnIntegerOverflow=on  OutDataTypeStr=Inherit: Same as input  ParamDataTypeStr=Inherit: Same as input
  pu : Gain  Gain=2/3*100  SaturateOnIntegerOverflow=on  OutDataTypeStr=Inherit: Same as input  ParamDataTypeStr=Inherit: Same as input
  pu->V : Gain  Gain=16e3*sqrt(2)  SaturateOnIntegerOverflow=on  OutDataTypeStr=Inherit: Same as input  ParamDataTypeStr=Inherit: Same as input
  pu1 : Gain  Gain=-1  SaturateOnIntegerOverflow=on  OutDataTypeStr=Inherit: Same as input  ParamDataTypeStr=Inherit: Same as input
  Va_Ia : Outport  VectorParamsAs1DForOutWhenUnconnected=off
  Q(Mvar) : Outport  Port=2  VectorParamsAs1DForOutWhenUnconnected=off
  "Vmeas Vref " : Outport  Port=3  VectorParamsAs1DForOutWhenUnconnected=off
  alpha TCR (deg) : Outport  Port=4  VectorParamsAs1DForOutWhenUnconnected=off
  nTSC : Outport  Port=5  VectorParamsAs1DForOutWhenUnconnected=off
  tag scope: I_TCRab=global, I_TSC1ab=global, I_TSC2ab=global, I_TSC3ab=global, Vab_Sec=global, Vc_TSC1ab=global, Vc_TSC2ab=global, Vc_TSC3ab=global
  wires:
  [TSC1_On] -> Mux/1
  [TSC2_On] -> Mux/2
  Mux/1 -> Data Type Conversion/1, Add/1
  [Vmeas] -> Mux1/1
  [Vref] -> Mux1/2
  [Vabc_Prim] -> Power (Positive-Sequence)/1, Selector3/1
  [Iabc_Prim] -> Power (Positive-Sequence)/2, Selector8/1
  Power (Positive-Sequence)/1 -> Terminator/1
  pu/1 -> pu1/1
  [BSVC] -> Controller Signals/2  "BSVC (pu/100MVA)"
  Mux1/1 -> Controller Signals/1, "Vmeas Vref "/1  "Vmeas Vref (pu)"
  [alpha] -> Controller Signals/3  "apha"
  Gain/1 -> Controller Signals/4  "TSC1 2 3"
  [TSC3_On] -> Mux/3
  Multimeter/1 -> A->pu1/1
  [TCRpulses] -> Selector2/1
  Selector2/1 -> TCRab/2  "Pulses AB + & -"
  Demux/1 -> [I_TCRab]
  Demux/4 -> [I_TSC3ab]
  [Vabc_Sec] -> Selector7/1
  Selector7/1 -> "V->pu "/1  "Vab Sec"
  [alpha] -> TCRab/3, alpha TCR (deg)/1  "alpha (deg)"
  [Vab_Sec] -> Mux2/1
  [I_TCRab] -> Mux2/2
  Mux2/1 -> TCRab/1  "Vab_sec (pu)  Iab_TCR (pu/100 MVA)"
  [Vab_Sec] -> Mux3/1
  [I_TSC1ab] -> Mux3/2
  Mux3/1 -> TSC2ab1/1  "Vab_sec (pu)  Iab_TSC1 (pu/100 MVA)"
  [TSC1pulses] -> Selector1/1
  "V->pu "/1 -> [Vab_Sec]
  Demux/2 -> [I_TSC1ab]
  Demux/3 -> [I_TSC2ab]
  Multimeter1/1 -> V->pu1/1
  Demux1/1 -> [Vc_TSC1ab]
  Demux1/2 -> [Vc_TSC2ab]
  Demux1/3 -> [Vc_TSC3ab]
  [Vc_TSC1ab] -> TSC2ab1/2  "Vab_C_TSC1 (pu)"
  [Vab_Sec] -> Mux4/1
  [I_TSC2ab] -> Mux4/2
  Mux4/1 -> TSC2ab/1  "Vab_sec (pu)  Iab_TSC2 (pu/100 MVA)"
  [TSC2pulses] -> Selector5/1
  [Vc_TSC2ab] -> TSC2ab/2  "Vab_C_TSC2 (pu)"
  Selector5/1 -> TSC2ab/3  "Pulses AB + & -"
  [Vab_Sec] -> Mux5/1
  [I_TSC3ab] -> Mux5/2
  Mux5/1 -> TSC3ab/1  "Vab_sec (pu)  Iab_TSC3 (pu/100 MVA)"
  [TSC3pulses] -> Selector6/1
  [Vc_TSC3ab] -> TSC3ab/2  "Vab_C_TSC3 (pu)"
  Selector6/1 -> TSC3ab/3  "Pulses AB + & -"
  pu1/1 -> Q(Mvar)/1
  Add/1 -> nTSC/1
  Selector3/1 -> Mux6/1
  Selector8/1 -> Mux6/2
  Mux6/1 -> Va_Ia/1
  [Vab_Sec] -> Mux7/1
  Mux7/1 -> pu->V/1
  [TSC1pulses] -> Selector4/1
  Selector4/1 -> TSC1 Misfiring/4  "Pulses Th+ AB"
  A->pu1/1 -> Demux/1
  V->pu1/1 -> Demux1/1
  [Vc_TSC1ab] -> Mux7/2
  Multimeter2/1 -> TSC1 Misfiring/3  "Iab _TSC1 (A)"
  [Vth_TSC1ab] -> TSC1 Misfiring/2  "V Th+ TSC1ab"
  pu->V/1 -> TSC1 Misfiring/1  "Vab_sec (pu)  Vab_C_TSC1 (pu)"
  Selector1/1 -> TSC2ab1/3  "Pulses AB + & -"
  Power (Positive-Sequence)/2 -> pu/1
  Data Type Conversion/1 -> Gain/1

== system Hybrid2_modified/Solar Plant ==
  Current-Controlled Current Source- Scale panel current to Np parallel strings : fl_lib/Electrical/Electrical Sources/Current-Controlled Current Source  K=-1*(solarPlant.numParallelPanel-1)  i1_specify=off  i1_priority=None  i1=0 A  i1_nominal_specify=off  i1_nominal_value=1  i1_nominal_unit=A  i2_specify=off  i2_priority=None  i2=0 A  i2_nominal_specify=off  i2_nominal_value=1  i2_nominal_unit=A
      settings: InternalSimscapePortConfiguration="{\"Bottom\":[],\"Left\":[{\"id\":\"p1\",\"label\":\"+\",\"type\":\"foundation.electrical.electrical\"},{\"id\":\"head\",\"label\":\"\",\"type\":\"foundation.electrical.electrical\"}],\"Right\":[{\"id\":\"n1\",\"label\":\"-\",\"type\":\"foundation.electrical.electrical\"},{\"id\":\"tail\",\"label\":\"\",\"type\":\"foundation.electrical.electrical\"}],\"Top\":[]}"
  Solar Panel : Subsystem  mask(Solar Panel){}
      mask help: Models a solar panel using a parallel-connected sting of solar cells. The solar cell strings are modeled using a single Solar Cell block from the Simscape(TM) Electrical(TM) Sources library.
      mask Display: image('SolarPanelValidationIcon.jpg')
  Voltage-Controlled Voltage Source - Scale panel voltage to Ns series panel : fl_lib/Electrical/Electrical Sources/Voltage-Controlled Voltage Source  K=-1*(solarPlant.numSeriesPanel-1)  v1_specify=off  v1_priority=None  v1=0 V  v1_nominal_specify=off  v1_nominal_value=1  v1_nominal_unit=V  v2_specify=off  v2_priority=None  v2=0 V  v2_nominal_specify=off  v2_nominal_value=1  v2_nominal_unit=V
      settings: InternalSimscapePortConfiguration="{\"Bottom\":[],\"Left\":[{\"id\":\"p1\",\"label\":\"+\",\"type\":\"foundation.electrical.electrical\"},{\"id\":\"p2\",\"label\":\"+\",\"type\":\"foundation.electrical.electrical\"}],\"Right\":[{\"id\":\"n1\",\"label\":\"-\",\"type\":\"foundation.electrical.electrical\"},{\"id\":\"n2\",\"label\":\"-\",\"type\":\"foundation.electrical.electrical\"}],\"Top\":[]}"
  + : PMIOPort  Side=Right
  Irradiance : PMIOPort  Port=2  Side=Left
  - : PMIOPort  Port=3  Side=Right
  connections:
  Voltage-Controlled Voltage Source - Scale panel voltage to Ns series panel/RConn2 -- Voltage-Controlled Voltage Source - Scale panel voltage to Ns series panel/RConn1 -- Solar Panel/RConn1
  Voltage-Controlled Voltage Source - Scale panel voltage to Ns series panel/LConn1 -- Current-Controlled Current Source- Scale panel current to Np parallel strings/LConn2 -- -/RConn1 -- Solar Panel/RConn2
  Current-Controlled Current Source- Scale panel current to Np parallel strings/RConn1 -- Current-Controlled Current Source- Scale panel current to Np parallel strings/RConn2 -- +/RConn1
  Current-Controlled Current Source- Scale panel current to Np parallel strings/LConn1 -- Voltage-Controlled Voltage Source - Scale panel voltage to Ns series panel/LConn2
  Solar Panel/LConn1 -- Irradiance/RConn1

== system Hybrid2_modified/Subsystem ==
  i : Inport
  Data Type Conversion : DataTypeConversion  SaturateOnIntegerOverflow=off  RndMeth=Floor
  Simulink-PS Converter : nesl_utility/Simulink-PS Converter  PhysicalDomain=network_engine_domain  SubClassName=ps_input  LeftPortType=input  RightPortType=output  PseudoPeriodic=off  Frequencies=[]  NoiseDistribution=none  NoiseParameters=[]  Unit=1  AffineConversion=off  FilteringAndDerivatives=provide  SimscapeFilterOrder=1  InputFilterTimeConstant=0.001  UdotUserProvided=0
  o : PMIOPort  Side=Right
  wires:
  Data Type Conversion/1 -> Simulink-PS Converter/1
  i/1 -> Data Type Conversion/1
  connections:
  Simulink-PS Converter/RConn1 -- o/RConn1

== system Hybrid2_modified/TCR1 ==
  note: Firing pulses
  note: TCR
  P : Inport  PortDimensions=6
  Demux : Demux  Outputs=6
      settings: DisplayOption=none
  Lab : spsSeriesRLCBranchLib/Series RLC Branch  LConnTagsString=__new0  RConnTagsString=__new0  BranchType=RL  Resistance=Rtcr  Inductance=Ltcr  SetiL0=off  InitialCurrent=0  Capacitance=1.0  Setx0=off  InitialVoltage=0  Measurements=Branch current
  Lbc : spsSeriesRLCBranchLib/Series RLC Branch  LConnTagsString=__new0  RConnTagsString=__new0  BranchType=RL  Resistance=Rtcr  Inductance=Ltcr  SetiL0=off  InitialCurrent=0  Capacitance=1.0  Setx0=off  InitialVoltage=0  Measurements=None
  Lca : spsSeriesRLCBranchLib/Series RLC Branch  LConnTagsString=__new0  RConnTagsString=__new0  BranchType=RL  Resistance=Rtcr  Inductance=Ltcr  SetiL0=off  InitialCurrent=0  Capacitance=1.0  Setx0=off  InitialVoltage=0  Measurements=None
  ThAB+ : spsThyristorLib/Thyristor  Ron=Ron  Lon=0  Vf=Vf  IC=0  Rs=Rsnub  Cs=Csnub  Measurements=off
      settings: AttributesFormatString=\n
  ThAB- : spsThyristorLib/Thyristor  Ron=Ron  Lon=0  Vf=Vf  IC=0  Rs=inf  Cs=0  Measurements=off
      settings: AttributesFormatString=\n
  ThBC+ : spsThyristorLib/Thyristor  Ron=Ron  Lon=0  Vf=Vf  IC=0  Rs=Rsnub  Cs=Csnub  Measurements=off
      settings: AttributesFormatString=\n
  ThBC- : spsThyristorLib/Thyristor  Ron=Ron  Lon=0  Vf=Vf  IC=0  Rs=inf  Cs=0  Measurements=off
      settings: AttributesFormatString=\n
  ThCA+ : spsThyristorLib/Thyristor  Ron=Ron  Lon=0  Vf=Vf  IC=0  Rs=Rsnub  Cs=Csnub  Measurements=off
      settings: AttributesFormatString=\n
  ThCA- : spsThyristorLib/Thyristor  Ron=Ron  Lon=0  Vf=Vf  IC=0  Rs=inf  Cs=0  Measurements=off
      settings: AttributesFormatString=\n
  A : PMIOPort  Side=Left
  B : PMIOPort  Port=2  Side=Left
  C : PMIOPort  Port=3  Side=Left
  wires:
  P/1 -> Demux/1
  Demux/1 -> [Ap]
  Demux/2 -> [Am]
  Demux/3 -> [Bp]
  Demux/4 -> [Bm]
  Demux/5 -> [Cp]
  [Cp] -> ThCA+/1
  [Cm] -> ThCA-/1
  Demux/6 -> [Cm]
  [Bm] -> ThBC-/1
  [Bp] -> ThBC+/1
  [Am] -> ThAB-/1
  [Ap] -> ThAB+/1
  connections:
  ThAB-/LConn1 -- ThAB+/RConn1 -- Lab/LConn1
  ThAB+/LConn1 -- ThAB-/RConn1 -- Lca/RConn1 -- A/RConn1
  ThBC-/LConn1 -- Lbc/LConn1 -- ThBC+/RConn1
  Lab/RConn1 -- ThBC-/RConn1 -- ThBC+/LConn1 -- B/RConn1
  Lca/LConn1 -- ThCA-/LConn1 -- ThCA+/RConn1
  Lbc/RConn1 -- ThCA-/RConn1 -- ThCA+/LConn1 -- C/RConn1
